simulink model "Q1_SP_Half_Wave_Rectifier"  (R2018a)
settings: Solver=FixedStepDiscrete  StartTime=0.0  StopTime=0.06  FixedStep=SampleTime  RelTol=1e-3
undefined symbols (not defined in the file): SampleTime
libraries: powerlib x6, powerlib_meascontrol x2
settings Model: Creator=Emre Deniz  LastModifiedBy=Furkan

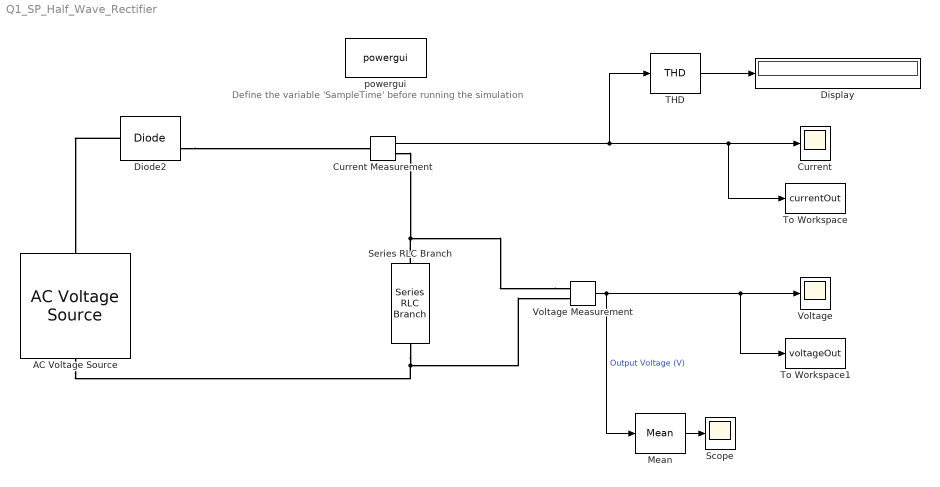
== system Q1_SP_Half_Wave_Rectifier ==
  note: Define the variable 'SampleTime' before running the simulation
  AC Voltage Source : powerlib/Electrical Sources/AC Voltage Source  Amplitude=230*sqrt(2)  Phase=0  Frequency=50  SampleTime=0  Measurements=Voltage  BusType=swing  Pref=10e3  Qref=0  Qmin=-inf  Qmax=+inf
  "Current " : Scope
  Current Measurement : powerlib/Measurements/Current Measurement  PhasorSimulation=off  OutputType=Complex  PSBequivalent=0
  Diode2 : powerlib/Power Electronics/Diode  Ron=1e-08  Lon=0  Vf=1e-6  IC=0  UseSnubber=0  Rs=0  Cs=0  Measurements=on
  Display : Display
      settings: Decimation=4
  Mean : powerlib_meascontrol/Measurements/Mean  Freq=50  Vinit=0  Ts=4e-3
  Scope : Scope
  Series RLC Branch : powerlib/Elements/Series RLC Branch  LConnTagsString=__new0  RConnTagsString=__new0  BranchType=R  Resistance=60  Inductance=0  SetiL0=off  InitialCurrent=0  Capacitance=0  Setx0=off  InitialVoltage=0  Measurements=None
  THD : powerlib_meascontrol/Measurements/THD  Freq=50  Ts=SampleTime
  To Workspace : ToWorkspace  VariableName=currentOut  SaveFormat=Structure With Time  SampleTime=-1
  To Workspace1 : ToWorkspace  VariableName=voltageOut  SaveFormat=Structure With Time  SampleTime=-1
  Voltage : Scope
  Voltage Measurement : powerlib/Measurements/Voltage Measurement  PhasorSimulation=off  OutputType=Complex  PSBequivalent=0
  powergui : powerlib/powergui  Priority=1  SimulationMode=Discrete  SampleTime=SampleTime  frequency=60  Iterations=50  frequencyindice=50  Pbase=100e6  ErrMax=1e-4  UnitsV=kV  UnitsW=MW  buscounter=0  FunctionMessages=off  echomessages=off  EnableUseOfTLC=off  CurrentSourceSwitches=off  DisableSnubberDevices=off  DisableRonSwitches=off  DisableVfSwitches=off  DisplayEquations=off  SolverType=Tustin/Backward Euler (TBE)  Interpol=off  ExternalGateDelay=off  methode=off  Ts=100  x0status=blocks  SPID=off  SwTol=0  HookPort=off  RestoreLinks=warning  ResistiveCurrentMeasurement=off  Frange=[0:2:500]  Ylog=off  Xlog=on  ShowGrid=off  save=off  variable=ZData  structure=currentOut  ZoomFFT=on  StartTime=0.0  cycles=1  DisplayStyle=3  fundamental=50  FreqAxis=on  MaxFrequency=1000  frequencyindicesteady=1  RmsSteady=1  display=off
  wires:
  Current Measurement/1 -> THD/1, To Workspace/1, "Current "/1
  Voltage Measurement/1 -> Mean/1, To Workspace1/1, Voltage/1  "Output Voltage (V)"
  Mean/1 -> Scope/1
  THD/1 -> Display/1
  connections:
  Series RLC Branch/RConn1 -- AC Voltage Source/LConn1 -- Voltage Measurement/LConn2
  Voltage Measurement/LConn1 -- Current Measurement/RConn1 -- Series RLC Branch/LConn1
  Diode2/RConn1 -- Current Measurement/LConn1
  Diode2/LConn1 -- AC Voltage Source/RConn1
